simulink model "Fmc"  (Simulink 8.4)
settings: Solver=ode45  StartTime=0.0  StopTime=10.0  RelTol=1e-3
undefined symbols (not defined in the file): Fmc_facKFuelMassCorr, Fmc_flgFuelMassCorrEnable, Fmc_flgFuelMassOverride, Fmc_mFuelMan, Fmc_tiTFuelMassCorr
settings Model: Creator=YAL9FE  LastModifiedBy=ric9fe
settings DebuggingCC: FcnCallInpInsideContextMsg=EnableAllAsWarning

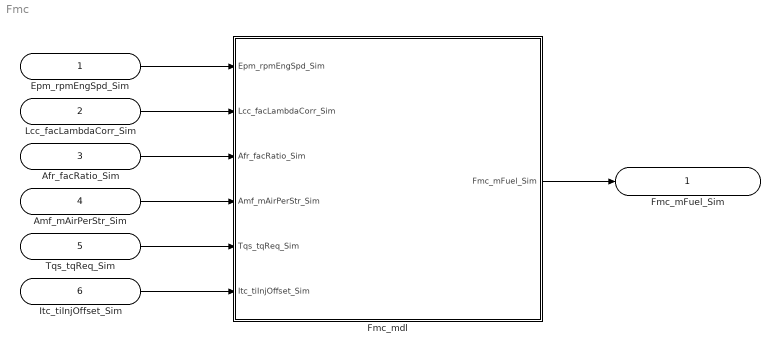
== system Fmc ==
  Epm_rpmEngSpd_Sim : Inport
  Lcc_facLambdaCorr_Sim : Inport  Port=2
  Afr_facRatio_Sim : Inport  Port=3
  Amf_mAirPerStr_Sim : Inport  Port=4
  Tqs_tqReq_Sim : Inport  Port=5
  Itc_tiInjOffset_Sim : Inport  Port=6
  Fmc_mdl : Subsystem  mask(Functions){}
      mask help: FuelMass
      mask Display:
      | image(imread('FuelMass.jpg'))
      | port_label('input',1,'Epm_rpmEngSpd_Sim')
      | port_label('input',2,'Lcc_facLambdaCorr_Sim')
      | port_label('input',3,'Afr_facRatio_Sim')
      | port_label('input',4,'Amf_mAirPerStr_Sim')
      | port_label('input',5,'Tqs_tqReq_Sim')
      | port_label('input',6,'Itc_tiInjOffset_Sim')
      | port_label('output',1,'Fmc_mFuel_Sim')
  Fmc_mFuel_Sim : Outport
  wires:
  Epm_rpmEngSpd_Sim/1 -> Fmc_mdl/1(Epm_rpmEngSpd_Sim)
  Lcc_facLambdaCorr_Sim/1 -> Fmc_mdl/2(Lcc_facLambdaCorr_Sim)
  Afr_facRatio_Sim/1 -> Fmc_mdl/3(Afr_facRatio_Sim)
  Amf_mAirPerStr_Sim/1 -> Fmc_mdl/4(Amf_mAirPerStr_Sim)
  Tqs_tqReq_Sim/1 -> Fmc_mdl/5(Tqs_tqReq_Sim)
  Itc_tiInjOffset_Sim/1 -> Fmc_mdl/6(Itc_tiInjOffset_Sim)
  Fmc_mdl/1(Fmc_mFuel_Sim) -> Fmc_mFuel_Sim/1

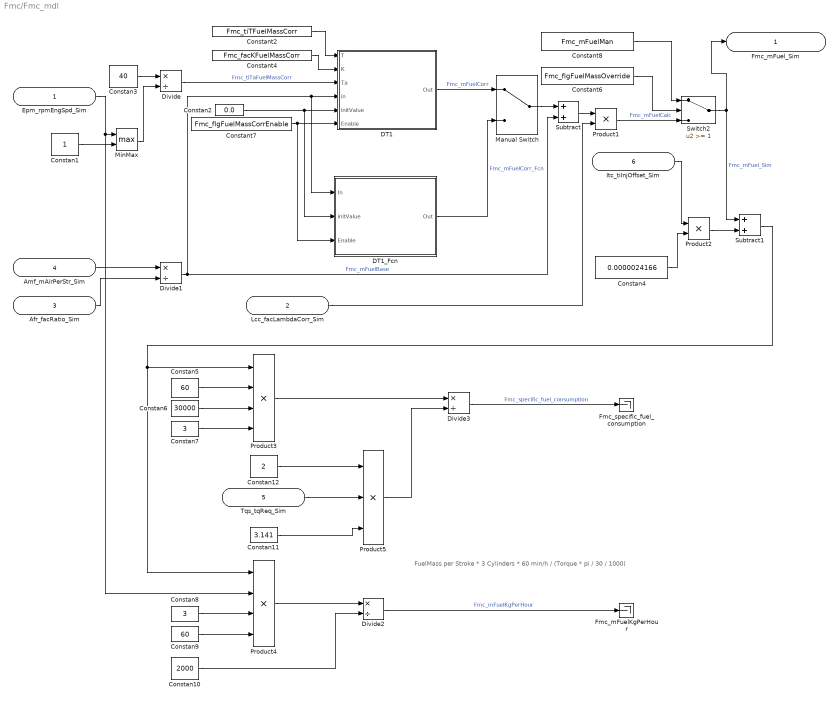
== system Fmc/Fmc_mdl ==
  note: FuelMass per Stroke * 3 Cylinders * 60 min/h / (Torque * pi / 30 / 1000)
  Epm_rpmEngSpd_Sim : Inport
  Lcc_facLambdaCorr_Sim : Inport  Port=2
  Afr_facRatio_Sim : Inport  Port=3
  Amf_mAirPerStr_Sim : Inport  Port=4
  Tqs_tqReq_Sim : Inport  Port=5
  Itc_tiInjOffset_Sim : Inport  Port=6
  Constan1 : Constant  OutDataTypeStr=single
  Constan10 : Constant  Value=2000  OutDataTypeStr=single
  Constan11 : Constant  Value=3.141  OutDataTypeStr=single
  Constan12 : Constant  Value=2  OutDataTypeStr=single
  Constan2 : Constant  Value=0.0  OutDataTypeStr=single
  Constan3 : Constant  Value=40  OutDataTypeStr=single
  Constan4 : Constant  Value=0.0000024166  OutDataTypeStr=single
  Constan5 : Constant  Value=60  OutDataTypeStr=single
  Constan6 : Constant  Value=30000  OutDataTypeStr=single
  Constan7 : Constant  Value=3  OutDataTypeStr=single
  Constan8 : Constant  Value=3  OutDataTypeStr=single
  Constan9 : Constant  Value=60  OutDataTypeStr=single
  Constant2 : Constant  Value=Fmc_tiTFuelMassCorr
  Constant4 : Constant  Value=Fmc_facKFuelMassCorr
  Constant6 : Constant  Value=Fmc_flgFuelMassOverride
  Constant7 : Constant  Value=Fmc_flgFuelMassCorrEnable
  Constant8 : Constant  Value=Fmc_mFuelMan
  DT1 : Subsystem
      mask help: DT1
      mask Display: image(imread('DT1.jpg'))
  DT1_Fcn : Subsystem
      mask help: DT1_Fcn
      mask Display: image(imread('DT1.jpg'))
  Divide{,1..3} (4 alike) : Product  Inputs=*/  OutDataTypeStr=Inherit: Same as first input
  Fmc_mFuelKgPerHour : Terminator
  Fmc_specific_fuel_consumption : Terminator
  Manual Switch : ManualSwitch
  MinMax : MinMax  Function=max  Inputs=2
  Product1 : Product  OutDataTypeStr=Inherit: Same as first input
  Product2 : Product  OutDataTypeStr=Inherit: Same as first input
  Product3 : Product  Inputs=4  OutDataTypeStr=Inherit: Same as first input
  Product4 : Product  Inputs=4  OutDataTypeStr=Inherit: Same as first input
  Product5 : Product  Inputs=3  OutDataTypeStr=Inherit: Same as first input
  Subtract : Sum  OutDataTypeStr=Inherit: Same as first input
  Subtract1 : Sum  OutDataTypeStr=Inherit: Same as first input
  Switch2 : Switch  Threshold=1
  Fmc_mFuel_Sim : Outport
  wires:
  Constant6/1 -> Switch2/2
  DT1/1(Out) -> Manual Switch/1  "Fmc_mFuelCorr"
  Constant2/1 -> DT1/1(T)
  Constant4/1 -> DT1/2(K)
  Constant7/1 -> DT1/6(Enable), DT1_Fcn/3(Enable)
  Constan3/1 -> Divide/1
  Divide/1 -> DT1/3(Ta)  "Fmc_tiTaFuelMassCorr"
  Constan2/1 -> DT1_Fcn/2(initValue), DT1/5(initValue)
  MinMax/1 -> Divide/2
  Epm_rpmEngSpd_Sim/1 -> MinMax/1, Product4/2
  Constan1/1 -> MinMax/2
  Amf_mAirPerStr_Sim/1 -> Divide1/1
  Afr_facRatio_Sim/1 -> Divide1/2
  Divide1/1 -> Subtract/2, DT1/4(in), DT1_Fcn/1(In)  "Fmc_mFuelBase"
  Constant8/1 -> Switch2/1
  Manual Switch/1 -> Subtract/1
  Subtract/1 -> Product1/1
  Lcc_facLambdaCorr_Sim/1 -> Product1/2
  Itc_tiInjOffset_Sim/1 -> Product2/1
  Product2/1 -> Subtract1/2
  Product1/1 -> Switch2/3  "Fmc_mFuelCalc"
  Switch2/1 -> Fmc_mFuel_Sim/1, Subtract1/1  "Fmc_mFuel_Sim"
  Constan4/1 -> Product2/2
  Subtract1/1 -> Product3/1, Product4/1
  Constan5/1 -> Product3/2
  Constan6/1 -> Product3/3
  Constan7/1 -> Product3/4
  Constan8/1 -> Product4/3
  Constan9/1 -> Product4/4
  Product4/1 -> Divide2/1
  Constan10/1 -> Divide2/2
  Constan12/1 -> Product5/1
  Tqs_tqReq_Sim/1 -> Product5/2
  Constan11/1 -> Product5/3
  Product3/1 -> Divide3/1
  Product5/1 -> Divide3/2
  Divide3/1 -> Fmc_specific_fuel_consumption/1  "Fmc_specific_fuel_consumption"
  Divide2/1 -> Fmc_mFuelKgPerHour/1  "Fmc_mFuelKgPerHour"
  DT1_Fcn/1(Out) -> Manual Switch/2  "Fmc_mFuelCorr_Fcn"

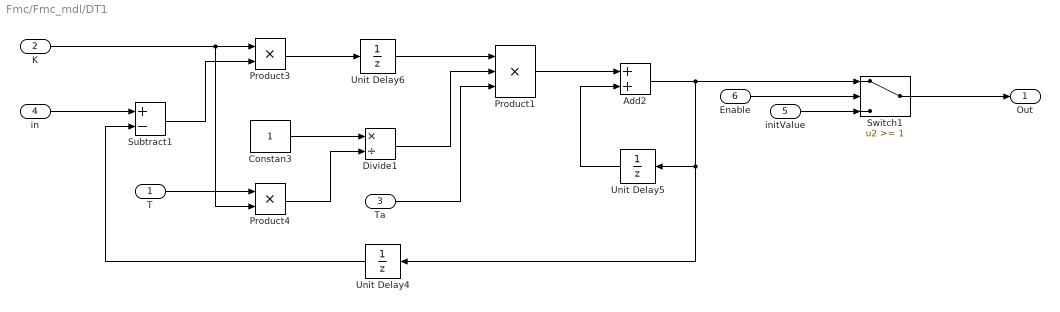
== system Fmc/Fmc_mdl/DT1 ==
  T : Inport
  K : Inport  Port=2
  Ta : Inport  Port=3
  in : Inport  Port=4
  initValue : Inport  Port=5
  Enable : Inport  Port=6
  Add2 : Sum  OutDataTypeStr=Inherit: Same as first input
  Constan3 : Constant  OutDataTypeStr=single
  Divide1 : Product  Inputs=*/  OutDataTypeStr=Inherit: Same as first input
  Product1 : Product  Inputs=3  OutDataTypeStr=Inherit: Same as first input
  Product3 : Product  OutDataTypeStr=Inherit: Same as first input
  Product4 : Product  OutDataTypeStr=Inherit: Same as first input
  Subtract1 : Sum  Inputs=+-
  Switch1 : Switch  Threshold=1
  Unit Delay4 : UnitDelay  SampleTime=-1
  Unit Delay5 : UnitDelay  SampleTime=-1
  Unit Delay6 : UnitDelay  SampleTime=-1
  Out : Outport
  wires:
  initValue/1 -> Switch1/3
  Switch1/1 -> Out/1
  in/1 -> Subtract1/1
  Subtract1/1 -> Product3/2
  K/1 -> Product3/1, Product4/2
  Product3/1 -> Unit Delay6/1
  Unit Delay6/1 -> Product1/1
  Constan3/1 -> Divide1/1
  T/1 -> Product4/1
  Product4/1 -> Divide1/2
  Divide1/1 -> Product1/2
  Product1/1 -> Add2/1
  Add2/1 -> Unit Delay5/1, Unit Delay4/1, Switch1/1
  Unit Delay5/1 -> Add2/2
  Unit Delay4/1 -> Subtract1/2
  Ta/1 -> Product1/3
  Enable/1 -> Switch1/2

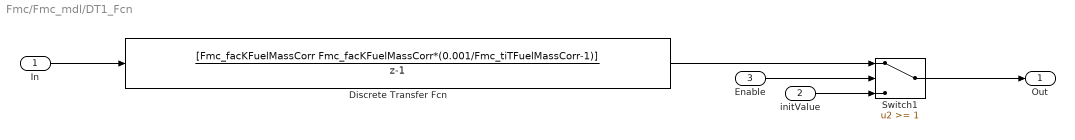
== system Fmc/Fmc_mdl/DT1_Fcn ==
  In : Inport
  initValue : Inport  Port=2
  Enable : Inport  Port=3
  Discrete Transfer Fcn : DiscreteTransferFcn  Numerator=[Fmc_facKFuelMassCorr Fmc_facKFuelMassCorr*(0.001/Fmc_tiTFuelMassCorr-1)]  Denominator=[1 -1]  OutDataTypeStr=Inherit: Same as input
  Switch1 : Switch  Threshold=1
  Out : Outport
  wires:
  In/1 -> Discrete Transfer Fcn/1
  initValue/1 -> Switch1/3
  Switch1/1 -> Out/1
  Discrete Transfer Fcn/1 -> Switch1/1
  Enable/1 -> Switch1/2
